simulink model "task"  (R2022b)
settings: Solver=VariableStepAuto  StartTime=0.0  StopTime=stoptime  RelTol=1e-9
values from neighbouring files (symbols this model uses):
  I = diag(I)    [taskmain.m]    (also in untitled.m = diag([1,1,1]))
  I_inv = pinv(I)    [taskmain.m]
  Ir = 0.005    [taskmain.m]
  k = [0;0;1]    [taskmain.m]
  M = [0;0;0]    [taskmain.m]
  Mr = 0    [taskmain.m]
  w0 = cat(1,w0,wr0)    [taskmain.m]
libraries: matrix_library x1
settings Model: Creator=a1pab  LastModifiedBy=a1pab

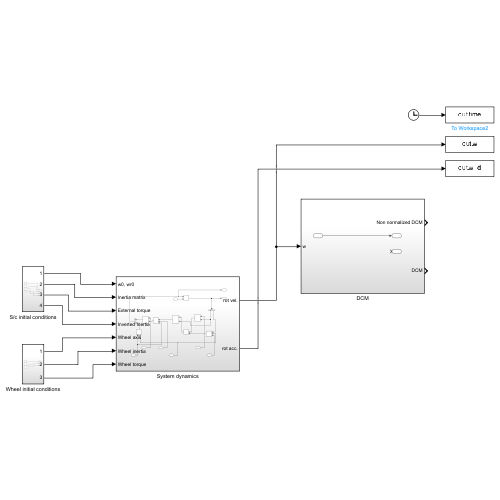
[thumbnail: Simulink's stored preview of the top-level diagram]
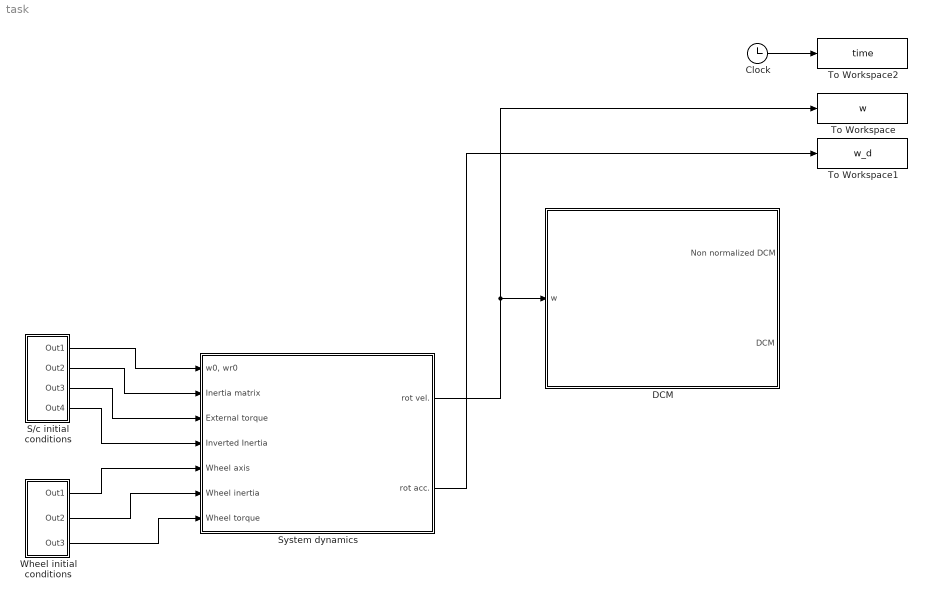
== system task ==
  Clock : Clock
  DCM : Subsystem
  S/c initial conditions : Subsystem
  System dynamics : Subsystem
  To Workspace : ToWorkspace  VariableName=w  SampleTime=-1
  To Workspace1 : ToWorkspace  VariableName=w_d  SampleTime=-1
  To Workspace2 : ToWorkspace  VariableName=time  SampleTime=-1
  Wheel initial conditions : Subsystem
  wires:
  System dynamics/1(rot vel.) -> DCM/1(w), To Workspace/1
  System dynamics/2(rot acc.) -> To Workspace1/1
  Clock/1 -> To Workspace2/1
  Wheel initial conditions/1(Out1) -> System dynamics/5(Wheel axis)
  Wheel initial conditions/2(Out2) -> System dynamics/6(Wheel inertia)
  Wheel initial conditions/3(Out3) -> System dynamics/7(Wheel torque)
  S/c initial conditions/1(Out1) -> System dynamics/1("w0, wr0")
  S/c initial conditions/2(Out2) -> System dynamics/2(Inertia matrix)
  S/c initial conditions/3(Out3) -> System dynamics/3(External torque)
  S/c initial conditions/4(Out4) -> System dynamics/4(Inverted Inertia)

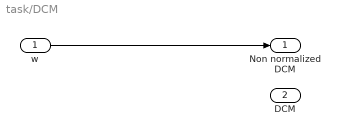
== system task/DCM ==
  w : Inport
  Non normalized DCM : Outport
  DCM : Outport  Port=2
  wires:
  w/1 -> Non normalized DCM/1

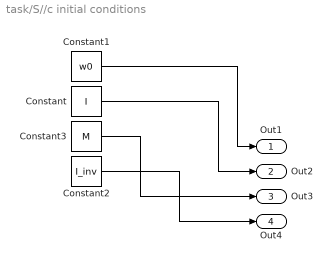
== system task/S//c initial conditions ==
  Constant : Constant  Value=I  VectorParams1D=off
  Constant1 : Constant  Value=w0  VectorParams1D=off
  Constant2 : Constant  Value=I_inv  VectorParams1D=off
  Constant3 : Constant  Value=M  VectorParams1D=off
  Out1 : Outport
  Out2 : Outport  Port=2
  Out3 : Outport  Port=3
  Out4 : Outport  Port=4
  wires:
  Constant3/1 -> Out3/1
  Constant1/1 -> Out1/1
  Constant2/1 -> Out4/1
  Constant/1 -> Out2/1

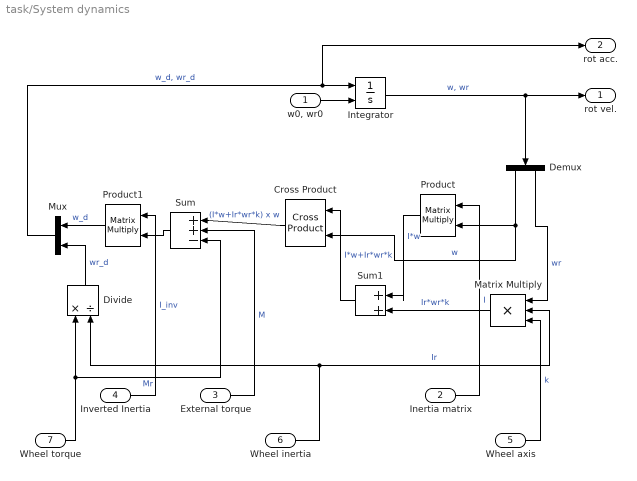
== system task/System dynamics ==
  "w0, wr0" : Inport
  Inertia matrix : Inport  Port=2
  External torque : Inport  Port=3
  Inverted Inertia : Inport  Port=4
  Wheel axis : Inport  Port=5
  Wheel inertia : Inport  Port=6
  Wheel torque : Inport  Port=7
  Cross Product : matrix_library/Cross Product
  Demux : Demux  Outputs=2
  Divide : Product  Inputs=*/
  Integrator : Integrator  InitialConditionSource=external
  Matrix Multiply : Product  Inputs=3
  Mux : Mux  Inputs=2
  Product : Product  Multiplication=Matrix(*)
  Product1 : Product  Multiplication=Matrix(*)
  Sum : Sum  Inputs=|++-
  Sum1 : Sum  Inputs=|++
  rot vel. : Outport
  rot acc. : Outport  Port=2
  wires:
  Mux/1 -> rot acc./1, Integrator/1  "w_d, wr_d"
  Integrator/1 -> Demux/1, rot vel./1  "w, wr"
  "w0, wr0"/1 -> Integrator/2
  Product/1 -> Sum1/1  "I*w"
  Cross Product/1 -> Sum/1  "(I*w+Ir*wr*k) x w"
  Inverted Inertia/1 -> Product1/1  "I_inv"
  Inertia matrix/1 -> Product/1  "I"
  Sum/1 -> Product1/2
  External torque/1 -> Sum/2  "M"
  Product1/1 -> Mux/1  "w_d"
  Wheel torque/1 -> Sum/3, Divide/1  "Mr"
  Wheel inertia/1 -> Matrix Multiply/2, Divide/2  "Ir"
  Divide/1 -> Mux/2  "wr_d"
  Demux/1 -> Cross Product/2, Product/2  "w"
  Sum1/1 -> Cross Product/1  "I*w+Ir*wr*k"
  Demux/2 -> Matrix Multiply/1  "wr"
  Matrix Multiply/1 -> Sum1/2  "Ir*wr*k"
  Wheel axis/1 -> Matrix Multiply/3  "k"

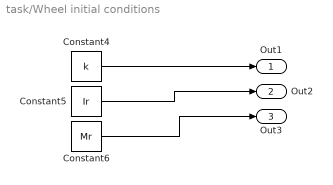
== system task/Wheel initial conditions ==
  Constant4 : Constant  Value=k  VectorParams1D=off
  Constant5 : Constant  Value=Ir
  Constant6 : Constant  Value=Mr
  Out1 : Outport
  Out2 : Outport  Port=2
  Out3 : Outport  Port=3
  wires:
  Constant4/1 -> Out1/1
  Constant5/1 -> Out2/1
  Constant6/1 -> Out3/1
